simulink model "pwaSys_reg_obs_model"  (Simulink 8.6)
settings: Solver=ode45  StartTime=0.0  StopTime=sim_T  RelTol=1e-3
InitFcn:
  | load simulink.mat
  | setParameters
StartFcn:
  | load simulink.mat
  | setParameters
  | clear res_X res_U res_Y res_P res_D
  | clear res_Xest res_Dest res_Yest
StopFcn:
  | plotScope
undefined symbols (not defined in the file or in its folder): sim_Cobs, sim_Dobs, sim_H, sim_K, sim_nd, sim_np, sim_nu, sim_nx, sim_ny, sim_x0
undefined symbols (not defined in the file): sim_A, sim_Aobs, sim_B, sim_Bobs, sim_C, sim_Cobs_fake, sim_D, sim_d0obs, sim_Dobs_fake, sim_Hobs, sim_Kobs, sim_TsObs, sim_x0obs
settings Model: Creator=alberto  LastModifiedBy=matteo
settings DataIOCC: SignalLoggingSaveFormat=Dataset
settings OptimizationCC: ExpressionDepthLimit=128
settings DebuggingCC: UnderspecifiedInitializationDetection=Simplified  MergeDetectMultiDrivingBlocksExec=error  FcnCallInpInsideContextMsg=EnableAllAsError  StateNameClashWarn=none
settings GRTTargetCC: CombineOutputUpdateFcns=on  GRTInterface=off
settings ConfigComp: CovSFcnEnable=off

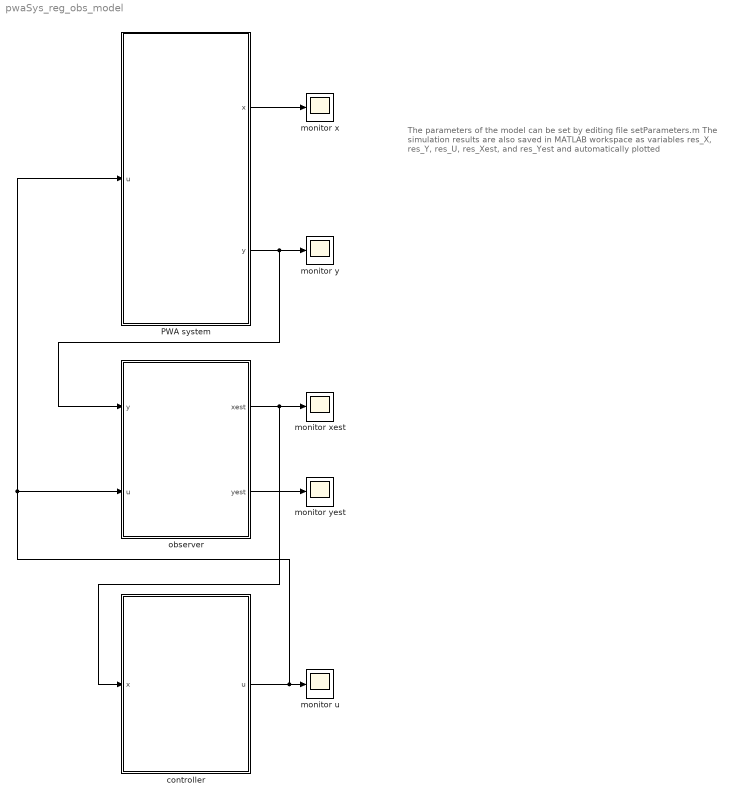
== system pwaSys_reg_obs_model ==
  note: The parameters of the model can be set by editing file setParameters.m
      |
      | The simulation results are also saved in MATLAB workspace as variables
      | res_X, res_Y, res_U, res_Xest, and res_Yest and automatically plotted
  PWA system : Subsystem
  controller : Subsystem
  monitor u : Scope
  monitor x : Scope
  monitor xest : Scope
  monitor y : Scope
  monitor yest : Scope
  observer : Subsystem
  wires:
  PWA system/1(x) -> monitor x/1
  PWA system/2(y) -> observer/1(y), monitor y/1
  observer/1(xest) -> monitor xest/1, controller/1(x)
  observer/2(yest) -> monitor yest/1
  controller/1(u) -> observer/2(u), PWA system/1(u), monitor u/1

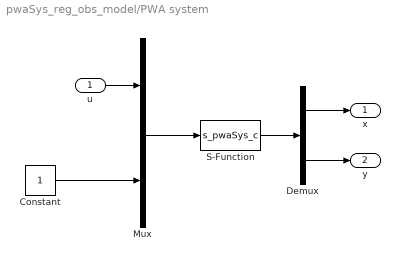
== system pwaSys_reg_obs_model/PWA system ==
  u : Inport
  Constant : Constant
  Demux : Demux  Outputs=[sim_nx sim_ny]
  Mux : Mux  Inputs=2
  S-Function : S-Function  FunctionName=s_pwaSys_c  Parameters=A,B,C,D,H,K,sim_x0  SFunctionDeploymentMode=off  EnableBusSupport=off  mask{A=sim_A, B=sim_B, C=sim_C, D=sim_D, H=sim_H, K=sim_K, sim_x0=sim_x0}
      mask prompts: sim_x0 "Initial condition"
      mask DialogControl DescTextVar Prompt: continuous time PWA system
  x : Outport
  y : Outport  Port=2
  wires:
  u/1 -> Mux/1
  Mux/1 -> S-Function/1
  S-Function/1 -> Demux/1
  Demux/1 -> x/1
  Demux/2 -> y/1
  Constant/1 -> Mux/2

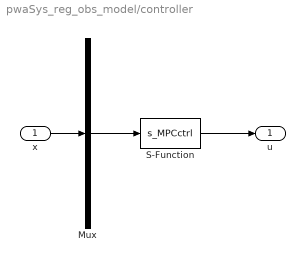
== system pwaSys_reg_obs_model/controller ==
  x : Inport
  Mux : Mux  Inputs=1
  S-Function : S-Function  FunctionName=s_MPCctrl  Parameters=sim_ctrl  SFunctionDeploymentMode=off  EnableBusSupport=off
  u : Outport
  wires:
  x/1 -> Mux/1
  Mux/1 -> S-Function/1
  S-Function/1 -> u/1

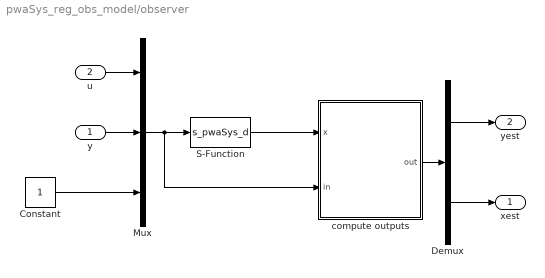
== system pwaSys_reg_obs_model/observer ==
  y : Inport
  u : Inport  Port=2
  Constant : Constant
  Demux : Demux  Outputs=[sim_ny sim_nx]
  Mux : Mux  Inputs=3
  S-Function : S-Function  FunctionName=s_pwaSys_d  Parameters=A,B,C,D,H,K,sim_x0,Ts  SFunctionDeploymentMode=off  EnableBusSupport=off  mask{A=sim_Aobs, B=sim_Bobs, C=sim_Cobs_fake, D=sim_Dobs_fake, H=sim_Hobs, K=sim_Kobs, sim_x0=[sim_x0obs;sim_d0obs], Ts=sim_TsObs}
      mask prompts: sim_x0 "Initial condition"; Ts "Sample time"
      mask DialogControl DescTextVar Prompt: continuous time PWA system
  compute outputs : Subsystem
  xest : Outport
  yest : Outport  Port=2
  wires:
  Mux/1 -> compute outputs/2(in), S-Function/1
  S-Function/1 -> compute outputs/1(x)
  Constant/1 -> Mux/3
  u/1 -> Mux/1
  Demux/1 -> yest/1
  Demux/2 -> xest/1
  compute outputs/1(out) -> Demux/1
  y/1 -> Mux/2

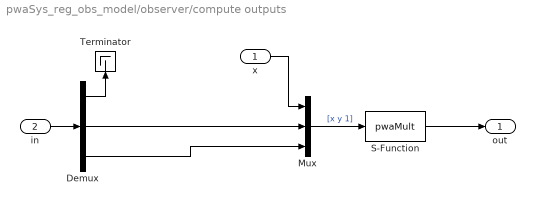
== system pwaSys_reg_obs_model/observer/compute outputs ==
  x : Inport
  in : Inport  Port=2
  Demux : Demux  Outputs=[sim_nu sim_ny 1]
  Mux : Mux  Inputs=3
  S-Function : S-Function  FunctionName=pwaMult  Parameters=sim_nx,sim_np,sim_nd,sim_nu,sim_H,sim_K,sim_Cobs,sim_Dobs  SFunctionDeploymentMode=off  EnableBusSupport=off
  Terminator : Terminator
  out : Outport
  wires:
  in/1 -> Demux/1
  Demux/2 -> Mux/2
  Demux/3 -> Mux/3
  Demux/1 -> Terminator/1
  x/1 -> Mux/1
  S-Function/1 -> out/1
  Mux/1 -> S-Function/1  "[x y 1]"
